simulink model "laneassist"  (R2020a)
settings: Solver=VariableStepAuto  StartTime=0.0  StopTime=10.0  RelTol=1e-3
undefined symbols (not defined in the file or in its folder): sigbuilder_block
libraries: simulink x1
settings Model: Creator=pc  LastModifiedBy=pc

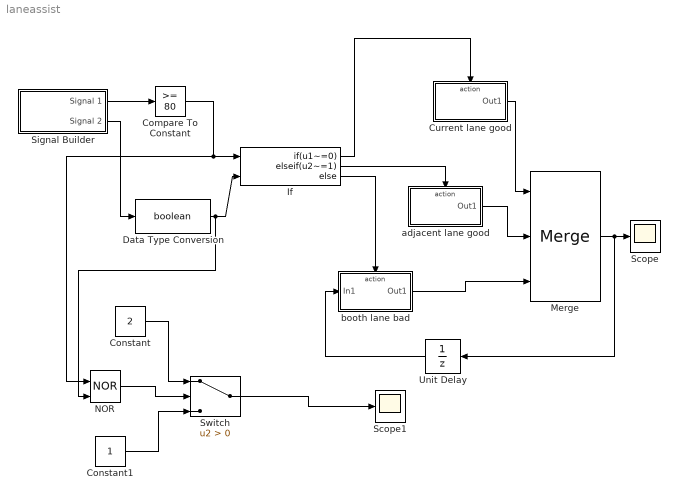
== system laneassist ==
  Compare To Constant : simulink/Logic and Bit Operations/Compare To Constant  relop=>=  const=80  OutDataTypeStr=boolean
  Constant : Constant  Value=2
  Constant1 : Constant
  Current lane good : Subsystem  TreatAsAtomicUnit=on
  Data Type Conversion : DataTypeConversion  OutDataTypeStr=boolean
  If : If  NumInputs=2  IfExpression=u1~=0  ElseIfExpressions=u2~=1
  Merge : Merge  Inputs=3
  NOR : Logic  Operator=NOR  IconShape=distinctive  AllPortsSameDT=off  OutDataTypeStr=boolean
  Scope : Scope
  Scope1 : Scope
  Signal Builder : Subsystem  Tag=STV Subsys  LoadFcn=sigbuilder_block('load');  StartFcn=sigbuilder_block('start');  StopFcn=sigbuilder_block('stop');  ClipboardFcn=sigbuilder_block('clipboard');  mask(Sigbuilder block){tuvar=[0:10]}
      mask help: Simulink:masks:SigbuilderBlock_MD
      mask init:
      | if ~strcmp(get_param(bdroot(gcbh),'SimulationStatus'),'stopped') tuvar = sigbuilder_block('maskInit'); end
      settings: CopyFcn=sigbuilder_block('copy');  DeleteFcn=sigbuilder_block('delete');  ModelCloseFcn=sigbuilder_block('modelClose');  PreSaveFcn=sigbuilder_block('preSave');  PauseFcn=sigbuilder_block('pause');  ContinueFcn=sigbuilder_block('continue');  NameChangeFcn=sigbuilder_block('namechange');  OpenFcn=sigbuilder_block('open',[97.5 51 550.5 359.25 ]);  CloseFcn=sigbuilder_block('close');
      mask Display: plot(0, 0, 100, 100,[2, 2, 32, 32, 2], [68, 8, 8, 68, 68],[32, 2], [38, 38], [32, 19, 2],[53, 60, 44], [32, 17, 17, 2],[16, 16, 31, 31]);txt = getActiveGroup(gcbh);text(2, 100, txt,'verticalAlignment', 'top');
  Switch : Switch  Criteria=u2 > Threshold
  Unit Delay : UnitDelay  SampleTime=-1  HasFrameUpgradeWarning=on
  adjacent lane good : Subsystem  TreatAsAtomicUnit=on
  booth lane bad : Subsystem  TreatAsAtomicUnit=on
  wires:
  If/1 -> Current lane good/Action
  If/2 -> adjacent lane good/Action
  If/3 -> booth lane bad/Action
  Signal Builder/1(Signal 1) -> Compare To Constant/1
  Compare To Constant/1 -> NOR/1, If/1
  Signal Builder/2(Signal 2) -> Data Type Conversion/1
  Data Type Conversion/1 -> NOR/2, If/2
  adjacent lane good/1(Out1) -> Merge/2
  booth lane bad/1(Out1) -> Merge/3
  Current lane good/1(Out1) -> Merge/1
  Merge/1 -> Unit Delay/1, Scope/1
  Unit Delay/1 -> booth lane bad/1(In1)
  Constant/1 -> Switch/1
  Constant1/1 -> Switch/3
  NOR/1 -> Switch/2
  Switch/1 -> Scope1/1

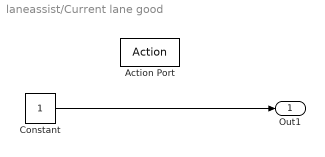
== system laneassist/Current lane good ==
  Action Port : ActionPort  ActionPortLabel=if(u1~=0)
  Constant : Constant
  Out1 : Outport
  wires:
  Constant/1 -> Out1/1

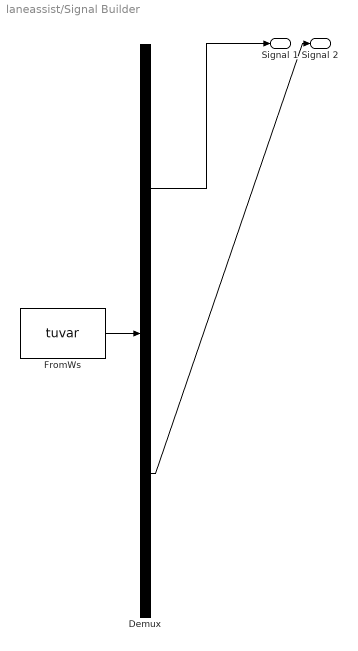
== system laneassist/Signal Builder ==
  Demux : Demux  Tag=STV Demux  Outputs=2
      settings: DisplayOption=none
  FromWs : FromWorkspace  Tag=STV FromWs  VariableName=tuvar
      SigBuilderData=|
      | common.afterFinalStr = 'Extrapolate'
      | common.sampleTime = 0
      | dataSet.timeRange = [0 10]
      | dataSet.name = 'Group 1'
      | sbobj.Groups.Name = 'Group 1'
      | sbobj.Groups.Signals(1).Name = 'Signal 1'
      | sbobj.Groups.Signals(1).XData = [0 4 4 6 6 10]
      | sbobj.Groups.Signals(1).YData = [80 80 50 50 80 80]
      | sbobj.Groups.Signals(2).Name = 'Signal 2'
      | sbobj.Groups.Signals(2).XData = [0 3 3 5 5 10]
      | sbobj.Groups.Signals(2).YData = [0 0 1 1 0 0]
  Signal 1 : Outport  Tag=STV Outport
  Signal 2 : Outport  Tag=STV Outport  Port=2
  wires:
  Demux/1 -> Signal 1/1
  FromWs/1 -> Demux/1
  Demux/2 -> Signal 2/1

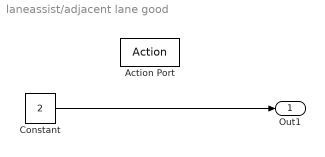
== system laneassist/adjacent lane good ==
  Action Port : ActionPort  ActionPortLabel=elseif(u2~=1)
  Constant : Constant  Value=2
  Out1 : Outport
  wires:
  Constant/1 -> Out1/1

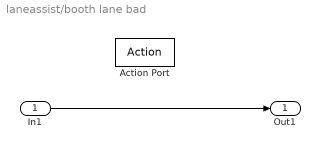
== system laneassist/booth lane bad ==
  In1 : Inport
  Action Port : ActionPort  ActionPortLabel=else
  Out1 : Outport
  wires:
  In1/1 -> Out1/1
